simulink model "Multicopter_vPC"  (R2017b)
settings: Solver=ode4  StartTime=0.0  StopTime=inf  FixedStep=0.0002  RelTol=1e-3
values from neighbouring files (symbols this model uses):
  ModelFailBatt_CustomHovTime = 15    [Init.m]
  ModelFailBatt_isEnable = boolean(0)    [Init.m]
  ModelFailBatt_islowCapacity = boolean(0)    [Init.m]
  ModelFailBatt_isLowVoltage = boolean(0)    [Init.m]
  ModelFailBatt_isPowOff = boolean(0)    [Init.m]
  ModelFailBatt_isUseCustomHovTime = boolean(0)    [Init.m]
  ModelFailBatt_remainCapacityRatio = 0.2    [Init.m]
  ModelFailBatt_remainVoltageRatio = 0.5    [Init.m]
  ModelFailEnable = boolean(0)    [Init.m]
  ModelFailLoad_isEnable = boolean(0)    [Init.m]
  ModelFailLoad_isLoadFall = boolean(0)    [Init.m]
  ModelFailLoad_isLoadLeak = boolean(0)    [Init.m]
  ModelFailLoad_isLoadShift = boolean(0)    [Init.m]
  ModelFailLoad_LoadLeakRatioRate = 0    [Init.m]
  ModelFailLoad_loadMassRatio = 0    [Init.m]
  ModelFailLoad_LoadShiftXRatio = 0    [Init.m]
  ModelFailLoad_LoadShiftYRatio = 0    [Init.m]
  ModelFailLoad_LoadShiftZRatio = 0    [Init.m]
  ModelFailProp_isEnable = boolean(1)    [Init.m]
  ModelFailProp_PropEffRatioVec = ones(1,8)    [Init.m]
  ModelFailWind_ConstWindX = 0    [Init.m]
  ModelFailWind_ConstWindY = 0    [Init.m]
  ModelFailWind_ConstWindZ = 0    [Init.m]
  ModelFailWind_GustWindFreq = 0    [Init.m]
  ModelFailWind_GustWindStrength = 0    [Init.m]
  ModelFailWind_isConstWind = boolean(0)    [Init.m]
  ModelFailWind_isEnable = boolean(0)    [Init.m]
  ModelFailWind_isGustWind = boolean(0)    [Init.m]
  ModelFailWind_isSheerWind = boolean(0)    [Init.m]
  ModelFailWind_isTurbWind = boolean(0)    [Init.m]
  ModelFailWind_SheerWindDirec = 0    [Init.m]
  ModelFailWind_SheerWindStrength = 0    [Init.m]
  ModelFailWind_TurbWindDirec = 0    [Init.m]
  ModelFailWind_TurbWindStrength = 0    [Init.m]
  ModelInit_RPM = 0    [Init.m]
  ModelParam_BattHoverMinutes = 18    [Init.m]
  ModelParam_BattHoverThr = 0.609    [Init.m]
  ModelParam_envAltitude = -41.5260009765625    (= -41.5260009766)    [Init.m]
  ModelParam_GlobalNoiseGainSwitch = 0    [Init.m]
  ModelParam_GPSEphFinal = 0.3    [Init.m]
  ModelParam_GPSEpvFinal = 0.4    [Init.m]
  ModelParam_GPSFix3DFix = 3    [Init.m]
  ModelParam_GPSSatsVisible = 10    [Init.m]
  ModelParam_motorCr = 1148    [Init.m]
  ModelParam_motorJm = 0.0001287    [Init.m]
  ModelParam_motorMinThr = 0.05    [Init.m]
  ModelParam_motorT = 0.02    [Init.m]
  ModelParam_motorWb = -141.4    [Init.m]
  ModelParam_noiseBaroCoupleWithSpeed = 0    [Init.m]
  ModelParam_noiseGPSSampTime = 0.2    [Init.m]
  ModelParam_noisePowerIMU = 0    [Init.m]
  ModelParam_noisePowerOffGainAccel = 0.04    [Init.m]
  ModelParam_noisePowerOffGainAccelZ = 0.03    [Init.m]
  ModelParam_noisePowerOffGainGyro = 0.02    [Init.m]
  ModelParam_noisePowerOffGainGyroZ = 0.025    [Init.m]
  ModelParam_noisePowerOffGainMag = 0.02    [Init.m]
  ModelParam_noisePowerOffGainMagZ = 0.035    [Init.m]
  ModelParam_noisePowerOnGainAccel = 0.8    [Init.m]
  ModelParam_noisePowerOnGainAccelZ = 4.5    [Init.m]
  ModelParam_noisePowerOnGainGyro = 2    [Init.m]
  ModelParam_noisePowerOnGainGyroZ = 1    [Init.m]
  ModelParam_noisePowerOnGainMag = 0.025    [Init.m]
  ModelParam_noisePowerOnGainMagZ = 0.05    [Init.m]
  ModelParam_noiseSampleTimeAccel = 0.001    [Init.m]
  ModelParam_noiseSampleTimeGyro = 0.001    [Init.m]
  ModelParam_noiseSampleTimeMag = 0.01    [Init.m]
  ModelParam_noiseUpperBaro = 0    [Init.m]
  ModelParam_noiseUpperGPS = 0.5    [Init.m]
  ModelParam_noiseUpperWindBodyRatio = 0    [Init.m]
  ModelParam_noiseWindSampTime = 0.001    [Init.m]
  ModelParam_rotorCm = 1.779e-07    [Init.m]
  ModelParam_rotorCt = 1.105e-05    [Init.m]
  ModelParam_timeSampBaro = 0.01    [Init.m]
  ModelParam_uavCCm = [0.0035 0.0039 0.0034]    [Init.m]
  ModelParam_uavCd = 0.055    [Init.m]
  ModelParam_uavDearo = 0.12    [Init.m]
  ModelParam_uavJ = [ModelParam_uavJxx,0,0;     0,ModelParam_uavJyy,0;     0,0,ModelParam_uavJzz]    [Init.m]
  ModelParam_uavMass = 1.4    [Init.m]
  ModelParam_uavMotNumbs = int8(4)    [Init.m]
  ModelParam_uavR = 0.225    [Init.m]
  ModelParam_uavType = int8(3)    [Init.m]
undefined symbols (not defined in the file or in its folder): d_i, Earth, F, h_i, Light, MIL, ModelParam_GPSEphInitial, ModelParam_GPSEphTimeConstant, ModelParam_GPSEpvInitial, ModelParam_GPSEpvTimeConstant, ModelParam_noiseLowPassFilterCoeAccel, ModelParam_noiseLowPassFilterCoeGyro, ModelParam_timeSamp, Moderate, Newton, Raphson, WGS84
libraries: simulink x12, aerolibasang x4, aerolibwind2 x3, aerolibtransform2 x3, sharedtransform x3, aerolibutil x2, sharedutil x2, shared6dof x1, aerolibatmos2 x1, aerolibconvert2 x1, aerolibobsolete x1, aerolibnav x1
(part 2 of 3)

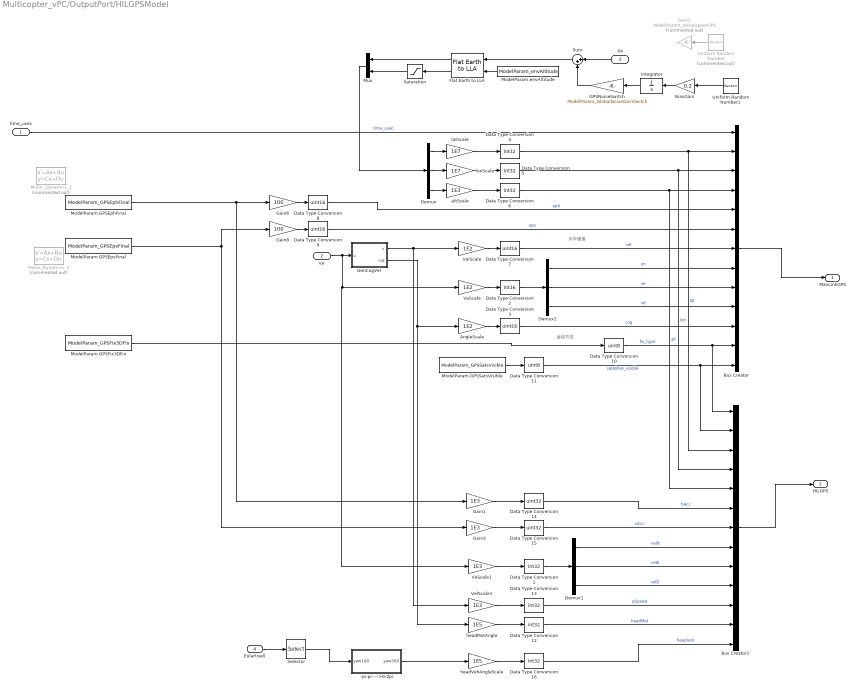
== system Multicopter_vPC/OutputPort/HILGPSModel ==
  note: 水平速度
  note: 运动方位
  time_usec : Inport
  Ve : Inport  Port=2
  Xe : Inport  Port=3
  Eular(rad) : Inport  Port=4
  -pi-pi---->0-2pi : MATLAB Function  TreatAsAtomicUnit=on
  AngleScale : Gain  Gain=1E2
  BiasGain : Gain  Gain=0.2
  Bus Creator : BusCreator  Inputs=13  OutDataTypeStr=Bus: MavLinkGPS  NonVirtualBus=on
  Bus Creator1 : BusCreator  Inputs=13  OutDataTypeStr=Bus: HILGPS  NonVirtualBus=on
  Data Type Conversion{1,4..6,12..13,16} (7 alike) : DataTypeConversion  OutDataTypeStr=int32
  Data Type Conversion10 : DataTypeConversion  OutDataTypeStr=uint8
  Data Type Conversion11 : DataTypeConversion  OutDataTypeStr=uint8
  Data Type Conversion14 : DataTypeConversion  OutDataTypeStr=uint32
  Data Type Conversion15 : DataTypeConversion  OutDataTypeStr=uint32
  Data Type Conversion2 : DataTypeConversion  OutDataTypeStr=int16
  Data Type Conversion{3,7..9} (4 alike) : DataTypeConversion  OutDataTypeStr=uint16
  Demux : Demux  Outputs=3
  Demux1 : Demux  Outputs=3
  Demux2 : Demux  Outputs=3
  Flat Earth to LLA : aerolibtransform2/Flat Earth to LLA  units=Metric (MKS)  ptype=Earth (WGS84)  F=1/298.257223563  R=6378137  LL0=ModelParam_GPSLatLong  psi=0
  GPSNoiseSwitch : Gain  Gain=ModelParam_GlobalNoiseGainSwitch
  Gain1 : Gain  Gain=1E3
  Gain2 : Gain  Commented=on  Gain=ModelParam_noiseUpperGPS
  Gain3 : Gain  Gain=1E3
  Gain6 : Gain  Gain=100
  Gain8 : Gain  Gain=100
  GenCogVel : MATLAB Function  TreatAsAtomicUnit=on
  Integrator : Integrator
  ModelParam.GPSEphFinal : Constant  Value=ModelParam_GPSEphFinal
  ModelParam.GPSEpvFinal : Constant  Value=ModelParam_GPSEpvFinal
  ModelParam.GPSFix3DFix : Constant  Value=ModelParam_GPSFix3DFix
  ModelParam.GPSSatsVisible : Constant  Value=ModelParam_GPSSatsVisible
  ModelParam.envAltitude : Constant  Value=ModelParam_envAltitude
  Motor_Dynamics_1 : StateSpace  Commented=on  A=-1/ModelParam_GPSEphTimeConstant  C=1/ModelParam_GPSEphTimeConstant  D=0  InitialCondition=ModelParam_GPSEphInitial*ModelParam_GPSEphTimeConstant
  Motor_Dynamics_2 : StateSpace  Commented=on  A=-1/ModelParam_GPSEpvTimeConstant  C=1/ModelParam_GPSEpvTimeConstant  D=0  InitialCondition=ModelParam_GPSEpvInitial*ModelParam_GPSEpvTimeConstant
  Mux : Mux  Inputs=2
  Saturation : Saturate  UpperLimit=100000  LowerLimit=0
  Selector : Selector  InputPortWidth=3  IndexOptions=Index vector (dialog)  Indices=[3]  OutputSizes=1
  Sum : Sum  Inputs=|++
  Uniform Random Number : UniformRandomNumber  Commented=on  Minimum=[-1,-1,-3]  Maximum=[1,1,3]  Seed=[14524,7875,698]  SampleTime=ModelParam_timeSamp
  Uniform Random Number1 : UniformRandomNumber  Minimum=[-1,-1,-1]  Maximum=[1,1,1]  Seed=[1452,787,69]  SampleTime=ModelParam_noiseGPSSampTime
  VeScale : Gain  Gain=1E2
  VeScale1 : Gain  Gain=1E3
  VelScale : Gain  Gain=1E2
  VelScale1 : Gain  Gain=1E3
  altScale : Gain  Gain=1E3
  headMotAngle : Gain  Gain=1E5
  headVehAngleScale : Gain  Gain=1E5
  latScale : Gain  Gain=1E7
  lonScale : Gain  Gain=1E7
  MavLinkGPS : Outport
  HILGPS : Outport  Port=2
  wires:
  Data Type Conversion16/1 -> Bus Creator1/13  "headVeh"
  headVehAngleScale/1 -> Data Type Conversion16/1
  Data Type Conversion12/1 -> Bus Creator1/12  "headMot"
  Data Type Conversion13/1 -> Bus Creator1/11  "gSpeed"
  Demux1/3 -> Bus Creator1/10  "velD"
  Demux1/2 -> Bus Creator1/9  "velE"
  Demux1/1 -> Bus Creator1/8  "velN"
  Data Type Conversion1/1 -> Demux1/1
  headMotAngle/1 -> Data Type Conversion12/1
  Data Type Conversion15/1 -> Bus Creator1/7  "vAcc"
  Data Type Conversion14/1 -> Bus Creator1/6  "hAcc"
  Gain3/1 -> Data Type Conversion15/1
  Gain1/1 -> Data Type Conversion14/1
  VeScale1/1 -> Data Type Conversion1/1
  VelScale1/1 -> Data Type Conversion13/1
  Data Type Conversion8/1 -> Bus Creator/5  "eph"
  Gain8/1 -> Data Type Conversion9/1
  Gain6/1 -> Data Type Conversion8/1
  Data Type Conversion9/1 -> Bus Creator/6  "epv"
  time_usec/1 -> Bus Creator/1  "time_usec"
  latScale/1 -> Data Type Conversion4/1
  lonScale/1 -> Data Type Conversion5/1
  altScale/1 -> Data Type Conversion6/1
  Data Type Conversion4/1 -> Bus Creator/2, Bus Creator1/3  "lat"
  Data Type Conversion5/1 -> Bus Creator/3, Bus Creator1/4  "lon"
  Data Type Conversion6/1 -> Bus Creator/4, Bus Creator1/5  "alt"
  Demux2/1 -> Bus Creator/8  "vn"
  Demux2/2 -> Bus Creator/9  "ve"
  Demux2/3 -> Bus Creator/10  "vd"
  VeScale/1 -> Data Type Conversion2/1
  Data Type Conversion2/1 -> Demux2/1
  VelScale/1 -> Data Type Conversion7/1
  Data Type Conversion7/1 -> Bus Creator/7  "vel"
  AngleScale/1 -> Data Type Conversion3/1
  Data Type Conversion3/1 -> Bus Creator/11  "cog"
  Data Type Conversion11/1 -> Bus Creator/13, Bus Creator1/2  "satellites_visible"
  Data Type Conversion10/1 -> Bus Creator/12, Bus Creator1/1  "fix_type"
  ModelParam.GPSSatsVisible/1 -> Data Type Conversion11/1
  Flat Earth to LLA/2 -> Saturation/1
  Saturation/1 -> Mux/2
  ModelParam.envAltitude/1 -> Flat Earth to LLA/2
  Xe/1 -> Sum/1
  Flat Earth to LLA/1 -> Mux/1
  Demux/1 -> latScale/1
  Demux/2 -> lonScale/1
  Demux/3 -> altScale/1
  Uniform Random Number/1 -> Gain2/1
  Sum/1 -> Flat Earth to LLA/1
  Uniform Random Number1/1 -> BiasGain/1
  Integrator/1 -> GPSNoiseSwitch/1
  BiasGain/1 -> Integrator/1
  Mux/1 -> Demux/1
  ModelParam.GPSEphFinal/1 -> Gain1/1, Gain6/1
  ModelParam.GPSEpvFinal/1 -> Gain8/1, Gain3/1
  ModelParam.GPSFix3DFix/1 -> Data Type Conversion10/1
  Ve/1 -> VeScale1/1, VeScale/1, GenCogVel/1(u)
  GenCogVel/1(v) -> VelScale/1, VelScale1/1
  GenCogVel/2(cot) -> AngleScale/1, headMotAngle/1
  Eular(rad)/1 -> Selector/1
  GPSNoiseSwitch/1 -> Sum/2
  Bus Creator/1 -> MavLinkGPS/1
  Bus Creator1/1 -> HILGPS/1
  -pi-pi---->0-2pi/1(yaw360) -> headVehAngleScale/1
  Selector/1 -> -pi-pi---->0-2pi/1(yaw180)

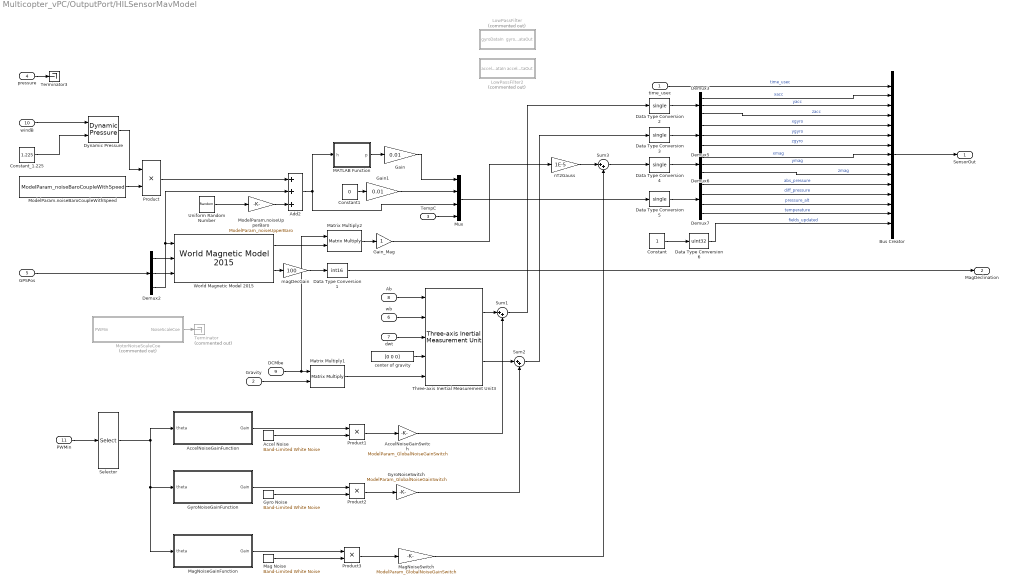
== system Multicopter_vPC/OutputPort/HILSensorMavModel ==
  time_usec : Inport
  Gravity : Inport  Port=2
  TempC : Inport  Port=3
  pressure : Inport  Port=4
  GPSPos : Inport  Port=5
  wb : Inport  Port=6
  dwt : Inport  Port=7
  Ab : Inport  Port=8
  DCMbe : Inport  Port=9
  windB : Inport  Port=10
  PWMin : Inport  Port=11
  Accel Noise : simulink/Sources/Band-Limited White Noise  Cov=ModelParam_noisePowerAccel  Ts=ModelParam_noiseSampleTimeAccel  seed=[411144,1416,71144]
  AccelNoiseGainFunction : MATLAB Function  TreatAsAtomicUnit=on
  AccelNoiseGainSwitch : Gain  Gain=ModelParam_GlobalNoiseGainSwitch
  Add2 : Sum  Inputs=+++
  Bus Creator : BusCreator  Inputs=15  OutDataTypeStr=Bus: MavLinkSensor  NonVirtualBus=on
  Constant : Constant
  Constant1 : Constant  Value=0
  Constant_1.225 : Constant  Value=1.225
  Data Type Conversion1 : DataTypeConversion  OutDataTypeStr=int16
  Data Type Conversion{2..5} (4 alike) : DataTypeConversion  OutDataTypeStr=single
  Data Type Conversion6 : DataTypeConversion  OutDataTypeStr=uint32
  Demux{2..3,5..6} (4 alike) : Demux  Outputs=3
  Demux7 : Demux
  Dynamic Pressure : aerolibasang/Dynamic Pressure
  Gain : Gain  Gain=0.01
  Gain1 : Gain  Gain=0.01
  Gain_Mag : Gain
  Gyro Noise : simulink/Sources/Band-Limited White Noise  Cov=ModelParam_noisePowerGyro  Ts=ModelParam_noiseSampleTimeGyro  seed=[111,116,144]
  GyroNoiseGainFunction : MATLAB Function  TreatAsAtomicUnit=on
  GyroNoiseSwitch : Gain  Gain=ModelParam_GlobalNoiseGainSwitch
  LowPassFilter : Subsystem  Commented=on
  LowPassFilter2 : Subsystem  Commented=on
  MATLAB Function : MATLAB Function  TreatAsAtomicUnit=on
  Mag Noise : simulink/Sources/Band-Limited White Noise  Cov=ModelParam_noisePowerMag  Ts=ModelParam_noiseSampleTimeMag  seed=[114,11699,999144]
  MagNoiseGainFunction : MATLAB Function  TreatAsAtomicUnit=on
  MagNoiseSwitch : Gain  Gain=ModelParam_GlobalNoiseGainSwitch
  Matrix Multiply1 : Product  Multiplication=Matrix(*)
  Matrix Multiply2 : Product  Multiplication=Matrix(*)
  ModelParam.noiseBaroCoupleWithSpeed : Constant  Value=ModelParam_noiseBaroCoupleWithSpeed
  ModelParam.noiseUpperBaro : Gain  Gain=ModelParam_noiseUpperBaro
  MotorNoiseScaleCoe : MATLAB Function  Commented=on  TreatAsAtomicUnit=on
  Mux : Mux
  Product{,1..3} (4 alike) : Product
  Selector : Selector  InputPortWidth=8  IndexOptions=Index vector (dialog)  Indices=[1]  OutputSizes=1
  Sum1 : Sum  Inputs=|++
  Sum2 : Sum  Inputs=|++
  Sum3 : Sum  Inputs=|++
  Terminator : Terminator  Commented=on
  Terminator3 : Terminator
  Three-axis Inertial Measurement Unit3 : aerolibnav/Three-axis Inertial Measurement Unit  units=Metric (MKS)  imu=[0 0 0]  i_Ts=0  dtype_a=on  w_a=190  z_a=0.707  a_sf_cc=[1 0 0; 0 1 0; 0 0 1]  a_bias=[0 0 0]  a_sat="[-160  -160  -160 160 160 160]"  dtype_g=on  w_g=190  z_g=0.707  g_sf_cc=[1 0 0; 0 1 0; 0 0 1]  g_bias=[0 0 0]  g_sens=[0 0 0]  g_sat="[-4.36  -4.36  -4.36 4.36 4.36 4.36]"  i_rand=off  i_seeds=[23093 23094 23095 23096 23097 23098]  i_pow=ModelParam_noisePowerIMU*[0.0000005 0.0000005 0.0000005 0.000000002 0.000000002 0.000000002]
  Uniform Random Number : UniformRandomNumber  Seed=15634  SampleTime=ModelParam_timeSampBaro
  World Magnetic Model 2015 : aerolibgravity2/World Magnetic Model 2015  units=Metric (MKS)  time_in=off  month=November  day=3  year=2017  action=Error  h_out=off  dec_out=on  inc_out=off  ti_out=off
      settings: SourceProductName=Aerospace Blockset  SourceProductBaseCode=AE
  center of gravity : Constant  Value=[0 0 0]
  magDecGain : Gain  Gain=100
  nT2Gauss : Gain  Gain=1E-5
  SensorOut : Outport
  MagDeclination : Outport  Port=2
  wires:
  center of gravity/1 -> Three-axis Inertial Measurement Unit3/4
  Sum1/1 -> Data Type Conversion2/1
  Sum2/1 -> Data Type Conversion3/1
  Sum3/1 -> Data Type Conversion4/1
  Matrix Multiply2/1 -> Gain_Mag/1
  magDecGain/1 -> Data Type Conversion1/1
  World Magnetic Model 2015/2 -> magDecGain/1
  ModelParam.noiseUpperBaro/1 -> Add2/3
  Product/1 -> Add2/1
  Dynamic Pressure/1 -> Product/1
  ModelParam.noiseBaroCoupleWithSpeed/1 -> Product/2
  Constant_1.225/1 -> Dynamic Pressure/2
  windB/1 -> Dynamic Pressure/1
  Uniform Random Number/1 -> ModelParam.noiseUpperBaro/1
  dwt/1 -> Three-axis Inertial Measurement Unit3/3
  Gain_Mag/1 -> nT2Gauss/1
  Constant1/1 -> Gain1/1
  pressure/1 -> Terminator3/1
  MATLAB Function/1(p) -> Gain/1
  Add2/1 -> MATLAB Function/1(h), Mux/3
  Demux2/3 -> World Magnetic Model 2015/1, Add2/2
  Demux2/2 -> World Magnetic Model 2015/3
  Demux2/1 -> World Magnetic Model 2015/2
  Matrix Multiply1/1 -> Three-axis Inertial Measurement Unit3/5
  DCMbe/1 -> Matrix Multiply2/1, Matrix Multiply1/1
  Gravity/1 -> Matrix Multiply1/2
  Gain1/1 -> Mux/2
  Gain/1 -> Mux/1
  Data Type Conversion6/1 -> Bus Creator/15  "fields_updated"
  Constant/1 -> Data Type Conversion6/1
  time_usec/1 -> Bus Creator/1  "time_usec"
  GPSPos/1 -> Demux2/1
  Demux7/2 -> Bus Creator/12  "diff_pressure"
  Demux7/3 -> Bus Creator/13  "pressure_alt"
  Demux6/2 -> Bus Creator/9  "ymag"
  Demux6/3 -> Bus Creator/10  "zmag"
  TempC/1 -> Mux/4
  Mux/1 -> Data Type Conversion5/1
  Demux7/1 -> Bus Creator/11  "abs_pressure"
  Demux5/2 -> Bus Creator/6  "ygyro"
  Demux6/1 -> Bus Creator/8  "xmag"
  Demux5/3 -> Bus Creator/7  "zgyro"
  Demux7/4 -> Bus Creator/14  "temperature"
  World Magnetic Model 2015/1 -> Matrix Multiply2/2
  Demux3/1 -> Bus Creator/2  "xacc"
  Demux3/2 -> Bus Creator/3  "yacc"
  Demux5/1 -> Bus Creator/5  "xgyro"
  Demux3/3 -> Bus Creator/4  "zacc"
  PWMin/1 -> Selector/1
  Ab/1 -> Three-axis Inertial Measurement Unit3/1
  wb/1 -> Three-axis Inertial Measurement Unit3/2
  MotorNoiseScaleCoe/1(NoiseScaleCoe) -> Terminator/1
  Selector/1 -> MagNoiseGainFunction/1(theta), GyroNoiseGainFunction/1(theta), AccelNoiseGainFunction/1(theta)
  AccelNoiseGainFunction/1(Gain) -> Product1/1
  GyroNoiseGainFunction/1(Gain) -> Product2/1
  Product1/1 -> AccelNoiseGainSwitch/1
  Product2/1 -> GyroNoiseSwitch/1
  Mag Noise/1 -> Product3/2
  nT2Gauss/1 -> Sum3/1
  Product3/1 -> MagNoiseSwitch/1
  MagNoiseGainFunction/1(Gain) -> Product3/1
  GyroNoiseSwitch/1 -> Sum2/2
  AccelNoiseGainSwitch/1 -> Sum1/2
  MagNoiseSwitch/1 -> Sum3/2
  Data Type Conversion2/1 -> Demux3/1
  Data Type Conversion3/1 -> Demux5/1
  Data Type Conversion4/1 -> Demux6/1
  Data Type Conversion5/1 -> Demux7/1
  Bus Creator/1 -> SensorOut/1
  Data Type Conversion1/1 -> MagDeclination/1
  Three-axis Inertial Measurement Unit3/1 -> Sum1/1
  Three-axis Inertial Measurement Unit3/2 -> Sum2/1
  Accel Noise/1 -> Product1/2
  Gyro Noise/1 -> Product2/2

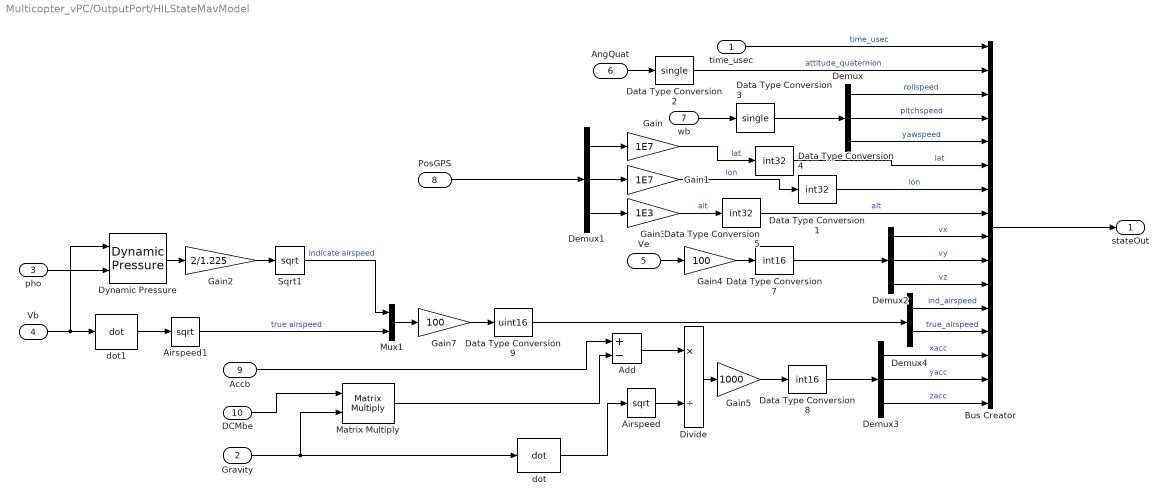
== system Multicopter_vPC/OutputPort/HILStateMavModel ==
  time_usec : Inport
  Gravity : Inport  Port=2
  pho : Inport  Port=3
  Vb : Inport  Port=4
  Ve : Inport  Port=5
  AngQuat : Inport  Port=6
  wb : Inport  Port=7
  PosGPS : Inport  Port=8
  Accb : Inport  Port=9
  DCMbe : Inport  Port=10
  Add : Sum  Inputs=+-
  Airspeed : Sqrt  AlgorithmType=Newton-Raphson  SaturateOnIntegerOverflow=on
  Airspeed1 : Sqrt  AlgorithmType=Newton-Raphson  SaturateOnIntegerOverflow=on
  Bus Creator : BusCreator  Inputs=16  OutDataTypeStr=Bus: MavLinkStateQuat  NonVirtualBus=on
  Data Type Conversion1 : DataTypeConversion  OutDataTypeStr=int32
  Data Type Conversion2 : DataTypeConversion  OutDataTypeStr=single
  Data Type Conversion3 : DataTypeConversion  OutDataTypeStr=single
  Data Type Conversion4 : DataTypeConversion  OutDataTypeStr=int32
  Data Type Conversion5 : DataTypeConversion  OutDataTypeStr=int32
  Data Type Conversion7 : DataTypeConversion  OutDataTypeStr=int16
  Data Type Conversion8 : DataTypeConversion  OutDataTypeStr=int16
  Data Type Conversion9 : DataTypeConversion  OutDataTypeStr=uint16
  Demux{,1..3} (4 alike) : Demux  Outputs=3
  Demux4 : Demux  Outputs=2
  Divide : Product  Inputs=*/
  Dynamic Pressure : aerolibasang/Dynamic Pressure
  Gain : Gain  Gain=1E7
  Gain1 : Gain  Gain=1E7
  Gain2 : Gain  Gain=2/1.225
  Gain3 : Gain  Gain=1E3
  Gain4 : Gain  Gain=100
  Gain5 : Gain  Gain=1000
  Gain7 : Gain  Gain=100
  Matrix Multiply : Product  Multiplication=Matrix(*)
  Mux1 : Mux  Inputs=2
  Sqrt1 : Sqrt  SaturateOnIntegerOverflow=on
  dot : aerolibasang/Incidence, Sideslip, & Airspeed/dot
      settings: SourceProductName=Aerospace Blockset  SourceProductBaseCode=AE
  dot1 : aerolibasang/Incidence, Sideslip, & Airspeed/dot
      settings: SourceProductName=Aerospace Blockset  SourceProductBaseCode=AE
  stateOut : Outport
  wires:
  Sqrt1/1 -> Mux1/1  "indicate airspeed"
  Gain2/1 -> Sqrt1/1
  Dynamic Pressure/1 -> Gain2/1
  time_usec/1 -> Bus Creator/1  "time_usec"
  Vb/1 -> dot1/1, Dynamic Pressure/1
  AngQuat/1 -> Data Type Conversion2/1
  Ve/1 -> Gain4/1
  Accb/1 -> Add/1
  wb/1 -> Data Type Conversion3/1
  Gravity/1 -> dot/1, Matrix Multiply/2
  Airspeed1/1 -> Mux1/2  "true airspeed"
  Mux1/1 -> Gain7/1
  Demux4/1 -> Bus Creator/12  "ind_airspeed"
  Demux4/2 -> Bus Creator/13  "true_airspeed"
  Demux3/3 -> Bus Creator/16  "zacc"
  Demux3/2 -> Bus Creator/15  "yacc"
  Demux3/1 -> Bus Creator/14  "xacc"
  Airspeed/1 -> Divide/2
  Gain5/1 -> Data Type Conversion8/1
  Divide/1 -> Gain5/1
  Demux2/3 -> Bus Creator/11  "vz"
  Demux2/2 -> Bus Creator/10  "vy"
  Demux2/1 -> Bus Creator/9  "vx"
  Gain4/1 -> Data Type Conversion7/1
  Gain3/1 -> Data Type Conversion5/1  "alt"
  Gain1/1 -> Data Type Conversion1/1  "lon"
  Gain/1 -> Data Type Conversion4/1  "lat"
  Demux1/3 -> Gain3/1
  Demux1/2 -> Gain1/1
  Demux1/1 -> Gain/1
  Demux/3 -> Bus Creator/5  "yawspeed"
  Demux/2 -> Bus Creator/4  "pitchspeed"
  Demux/1 -> Bus Creator/3  "rollspeed"
  Data Type Conversion2/1 -> Bus Creator/2  "attitude_quaternion"
  pho/1 -> Dynamic Pressure/2
  Gain7/1 -> Data Type Conversion9/1
  dot1/1 -> Airspeed1/1
  dot/1 -> Airspeed/1
  Data Type Conversion3/1 -> Demux/1
  PosGPS/1 -> Demux1/1
  Data Type Conversion7/1 -> Demux2/1
  Data Type Conversion9/1 -> Demux4/1
  Data Type Conversion8/1 -> Demux3/1
  Data Type Conversion4/1 -> Bus Creator/6  "lat"
  Data Type Conversion1/1 -> Bus Creator/7  "lon"
  Data Type Conversion5/1 -> Bus Creator/8  "alt"
  Bus Creator/1 -> stateOut/1
  DCMbe/1 -> Matrix Multiply/1
  Matrix Multiply/1 -> Add/2
  Add/1 -> Divide/1

== system Multicopter_vPC/Actuator Model: Motor_ESC/MotorNonlinearDynamic1/Motor_Dynamics ==
  motor_rate_d : Inport
  ModelInit_RPM : Inport  Port=2
  motorT : Inport  Port=3
  Add : Sum  Inputs=+-
  Divide : Product  Inputs=*/
  Integrator : Integrator  InitialConditionSource=external
  motor_rate_act : Outport
  wires:
  motorT/1 -> Divide/2
  Integrator/1 -> Add/2, motor_rate_act/1  "x"
  Divide/1 -> Integrator/1  "drate/dt"
  motor_rate_d/1 -> Add/1
  ModelInit_RPM/1 -> Integrator/2
  Add/1 -> Divide/1

== system Multicopter_vPC/Actuator Model: Motor_ESC/MotorNonlinearDynamic2/Motor_Dynamics ==
  motor_rate_d : Inport
  ModelInit_RPM : Inport  Port=2
  motorT : Inport  Port=3
  Add : Sum  Inputs=+-
  Divide : Product  Inputs=*/
  Integrator : Integrator  InitialConditionSource=external
  motor_rate_act : Outport
  wires:
  Add/1 -> Divide/1
  ModelInit_RPM/1 -> Integrator/2
  motor_rate_d/1 -> Add/1
  Divide/1 -> Integrator/1  "drate/dt"
  Integrator/1 -> motor_rate_act/1, Add/2  "x"
  motorT/1 -> Divide/2

== system Multicopter_vPC/Actuator Model: Motor_ESC/MotorNonlinearDynamic3/Motor_Dynamics ==
  motor_rate_d : Inport
  ModelInit_RPM : Inport  Port=2
  motorT : Inport  Port=3
  Add : Sum  Inputs=+-
  Divide : Product  Inputs=*/
  Integrator : Integrator  InitialConditionSource=external
  motor_rate_act : Outport
  wires:
  motorT/1 -> Divide/2
  Integrator/1 -> Add/2, motor_rate_act/1  "x"
  Divide/1 -> Integrator/1  "drate/dt"
  motor_rate_d/1 -> Add/1
  ModelInit_RPM/1 -> Integrator/2
  Add/1 -> Divide/1

== system Multicopter_vPC/Actuator Model: Motor_ESC/MotorNonlinearDynamic4/Motor_Dynamics ==
  motor_rate_d : Inport
  ModelInit_RPM : Inport  Port=2
  motorT : Inport  Port=3
  Add : Sum  Inputs=+-
  Divide : Product  Inputs=*/
  Integrator : Integrator  InitialConditionSource=external
  motor_rate_act : Outport
  wires:
  Add/1 -> Divide/1
  ModelInit_RPM/1 -> Integrator/2
  motor_rate_d/1 -> Add/1
  Divide/1 -> Integrator/1  "drate/dt"
  Integrator/1 -> motor_rate_act/1, Add/2  "x"
  motorT/1 -> Divide/2

== system Multicopter_vPC/Actuator Model: Motor_ESC/MotorNonlinearDynamic5/Motor_Dynamics ==
  motor_rate_d : Inport
  ModelInit_RPM : Inport  Port=2
  motorT : Inport  Port=3
  Add : Sum  Inputs=+-
  Divide : Product  Inputs=*/
  Integrator : Integrator  InitialConditionSource=external
  motor_rate_act : Outport
  wires:
  motorT/1 -> Divide/2
  Integrator/1 -> Add/2, motor_rate_act/1  "x"
  Divide/1 -> Integrator/1  "drate/dt"
  motor_rate_d/1 -> Add/1
  ModelInit_RPM/1 -> Integrator/2
  Add/1 -> Divide/1

== system Multicopter_vPC/Actuator Model: Motor_ESC/MotorNonlinearDynamic6/Motor_Dynamics ==
  motor_rate_d : Inport
  ModelInit_RPM : Inport  Port=2
  motorT : Inport  Port=3
  Add : Sum  Inputs=+-
  Divide : Product  Inputs=*/
  Integrator : Integrator  InitialConditionSource=external
  motor_rate_act : Outport
  wires:
  Add/1 -> Divide/1
  ModelInit_RPM/1 -> Integrator/2
  motor_rate_d/1 -> Add/1
  Divide/1 -> Integrator/1  "drate/dt"
  Integrator/1 -> motor_rate_act/1, Add/2  "x"
  motorT/1 -> Divide/2

== system Multicopter_vPC/Actuator Model: Motor_ESC/MotorNonlinearDynamic7/Motor_Dynamics ==
  motor_rate_d : Inport
  ModelInit_RPM : Inport  Port=2
  motorT : Inport  Port=3
  Add : Sum  Inputs=+-
  Divide : Product  Inputs=*/
  Integrator : Integrator  InitialConditionSource=external
  motor_rate_act : Outport
  wires:
  motorT/1 -> Divide/2
  Integrator/1 -> Add/2, motor_rate_act/1  "x"
  Divide/1 -> Integrator/1  "drate/dt"
  motor_rate_d/1 -> Add/1
  ModelInit_RPM/1 -> Integrator/2
  Add/1 -> Divide/1

== system Multicopter_vPC/Actuator Model: Motor_ESC/MotorNonlinearDynamic8/Motor_Dynamics ==
  motor_rate_d : Inport
  ModelInit_RPM : Inport  Port=2
  motorT : Inport  Port=3
  Add : Sum  Inputs=+-
  Divide : Product  Inputs=*/
  Integrator : Integrator  InitialConditionSource=external
  motor_rate_act : Outport
  wires:
  Add/1 -> Divide/1
  ModelInit_RPM/1 -> Integrator/2
  motor_rate_d/1 -> Add/1
  Divide/1 -> Integrator/1  "drate/dt"
  Integrator/1 -> motor_rate_act/1, Add/2  "x"
  motorT/1 -> Divide/2

== system Multicopter_vPC/Force and Moment Model/Propeller Model/Multicopter ==
  uavType : Inport
  MotorRads : Inport  Port=2
  uavR : Inport  Port=3
  uavDearo : Inport  Port=4
  Cm : Inport  Port=5
  Ct : Inport  Port=6
  Jm : Inport  Port=7
  wb : Inport  Port=8
  Action Port : ActionPort  InitializeStates=reset
  For Iterator Subsystem : Subsystem  TreatAsAtomicUnit=on
  Gain : Gain  Gain=-1
  Vector Concatenate : Concatenate
  Vector Concatenate1 : Concatenate  NumInputs=3  Mode=Multidimensional array
  uavTypeDefine : MATLAB Function  TreatAsAtomicUnit=on
  Fb : Outport
  Mb : Outport  Port=2
  wires:
  wb/1 -> For Iterator Subsystem/2(wb)
  uavR/1 -> Vector Concatenate/1
  uavDearo/1 -> Gain/1
  Gain/1 -> Vector Concatenate/2
  Vector Concatenate/1 -> For Iterator Subsystem/4(motorPositionVector)
  MotorRads/1 -> For Iterator Subsystem/5(motorOmegaVector)
  Cm/1 -> For Iterator Subsystem/9(rotorCm)
  Ct/1 -> For Iterator Subsystem/8(rotorCt)
  Jm/1 -> For Iterator Subsystem/6(motorJ_RP)
  For Iterator Subsystem/2(Mb) -> Mb/1
  For Iterator Subsystem/1(Fb) -> Fb/1
  uavType/1 -> uavTypeDefine/1(uavType)
  uavTypeDefine/1(n_p) -> For Iterator Subsystem/1(n_p)
  uavTypeDefine/5(motorRotateDirectionVector) -> For Iterator Subsystem/7(motorRotateDirectionVector)
  uavTypeDefine/4(motorPsiVector) -> Vector Concatenate1/3
  uavTypeDefine/3(motorThetaVector) -> Vector Concatenate1/2
  uavTypeDefine/2(motorPhiVector) -> Vector Concatenate1/1
  Vector Concatenate1/1 -> For Iterator Subsystem/3(motorEularMatrix)

== system Multicopter_vPC/Force and Moment Model/Propeller Model/Other Vehicle Types ==
  MotorRads : Inport
  Action Port : ActionPort  InitializeStates=reset
  Constant : Constant  Value=[0,0,0]
  Constant1 : Constant  Value=[0,0,0]
  Terminator : Terminator
  Fb : Outport
  Mb : Outport  Port=2
  wires:
  Constant/1 -> Fb/1
  Constant1/1 -> Mb/1
  MotorRads/1 -> Terminator/1

== system Multicopter_vPC/OutputPort/HILSensorMavModel/LowPassFilter ==
  gyroDataIn : Inport
  Demux1 : Demux  Outputs=3
  Mux1 : Mux  Inputs=3
  x : TransferFcn  Denominator=[ModelParam_noiseLowPassFilterCoeGyro 1]
  y : TransferFcn  Denominator=[ModelParam_noiseLowPassFilterCoeGyro 1]
  z : TransferFcn  Denominator=[ModelParam_noiseLowPassFilterCoeGyro 1]
  gyroDataOut : Outport
  wires:
  Mux1/1 -> gyroDataOut/1
  z/1 -> Mux1/3
  x/1 -> Mux1/1
  Demux1/1 -> x/1
  y/1 -> Mux1/2
  gyroDataIn/1 -> Demux1/1
  Demux1/2 -> y/1
  Demux1/3 -> z/1

== system Multicopter_vPC/OutputPort/HILSensorMavModel/LowPassFilter2 ==
  accelDataIn : Inport
  Demux1 : Demux  Outputs=3
  Mux1 : Mux  Inputs=3
  x : TransferFcn  Denominator=[ModelParam_noiseLowPassFilterCoeAccel 1]
  y : TransferFcn  Denominator=[ModelParam_noiseLowPassFilterCoeAccel 1]
  z : TransferFcn  Denominator=[ModelParam_noiseLowPassFilterCoeAccel 1]
  accelDataOut : Outport
  wires:
  Mux1/1 -> accelDataOut/1
  z/1 -> Mux1/3
  x/1 -> Mux1/1
  Demux1/1 -> x/1
  y/1 -> Mux1/2
  accelDataIn/1 -> Demux1/1
  Demux1/2 -> y/1
  Demux1/3 -> z/1

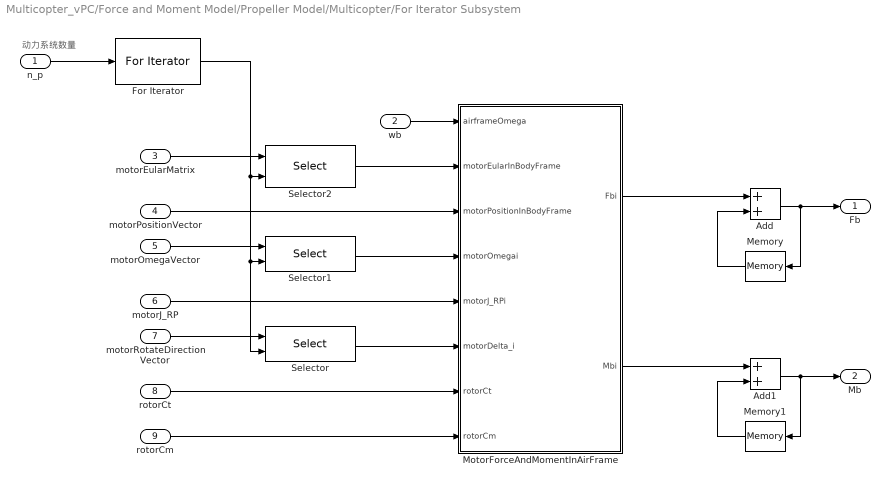
== system Multicopter_vPC/Force and Moment Model/Propeller Model/Multicopter/For Iterator Subsystem ==
  note: 动力系统数量
  n_p : Inport
  wb : Inport  Port=2
  motorEularMatrix : Inport  Port=3
  motorPositionVector : Inport  Port=4
  motorOmegaVector : Inport  Port=5
  motorJ_RP : Inport  Port=6
  motorRotateDirectionVector : Inport  Port=7
  rotorCt : Inport  Port=8
  rotorCm : Inport  Port=9
  Add : Sum
  Add1 : Sum
  For Iterator : ForIterator  ResetStates=reset  IterationSource=external
  Memory : Memory  InitialCondition=[0;0;0]  InheritSampleTime=on
  Memory1 : Memory  InitialCondition=[0;0;0]  InheritSampleTime=on
  MotorForceAndMomentInAirFrame : Subsystem  mask(Multicopter_Force_and_Moment_Model){}
      mask help: 在模块上右键帮助,查看帮助文档
      mask Help: web('doc/Multicopter_Force_and_Moment_Model.html')
  Selector : Selector  InputPortWidth=8  IndexOptions=Index vector (port)  Indices=[1 3]  OutputSizes=1
  Selector1 : Selector  InputPortWidth=8  IndexOptions=Index vector (port)  Indices=[1 3]  OutputSizes=1
  Selector2 : Selector  NumberOfDimensions=2  InputPortWidth=8  IndexOptions=Select all,Index vector (port)  Indices=[1 3],1  OutputSizes=1,1
  Fb : Outport
  Mb : Outport  Port=2
  wires:
  n_p/1 -> For Iterator/1
  wb/1 -> MotorForceAndMomentInAirFrame/1(airframeOmega)
  motorPositionVector/1 -> MotorForceAndMomentInAirFrame/3(motorPositionInBodyFrame)
  rotorCm/1 -> MotorForceAndMomentInAirFrame/8(rotorCm)
  rotorCt/1 -> MotorForceAndMomentInAirFrame/7(rotorCt)
  motorJ_RP/1 -> MotorForceAndMomentInAirFrame/5(motorJ_RPi)
  For Iterator/1 -> Selector2/2, Selector1/2, Selector/2
  motorRotateDirectionVector/1 -> Selector/1
  Selector/1 -> MotorForceAndMomentInAirFrame/6(motorDelta_i)
  Selector1/1 -> MotorForceAndMomentInAirFrame/4(motorOmegai)
  motorOmegaVector/1 -> Selector1/1
  Selector2/1 -> MotorForceAndMomentInAirFrame/2(motorEularInBodyFrame)
  motorEularMatrix/1 -> Selector2/1
  MotorForceAndMomentInAirFrame/1(Fbi) -> Add/1
  Memory/1 -> Add/2
  Add/1 -> Fb/1, Memory/1
  MotorForceAndMomentInAirFrame/2(Mbi) -> Add1/1
  Memory1/1 -> Add1/2
  Add1/1 -> Mb/1, Memory1/1

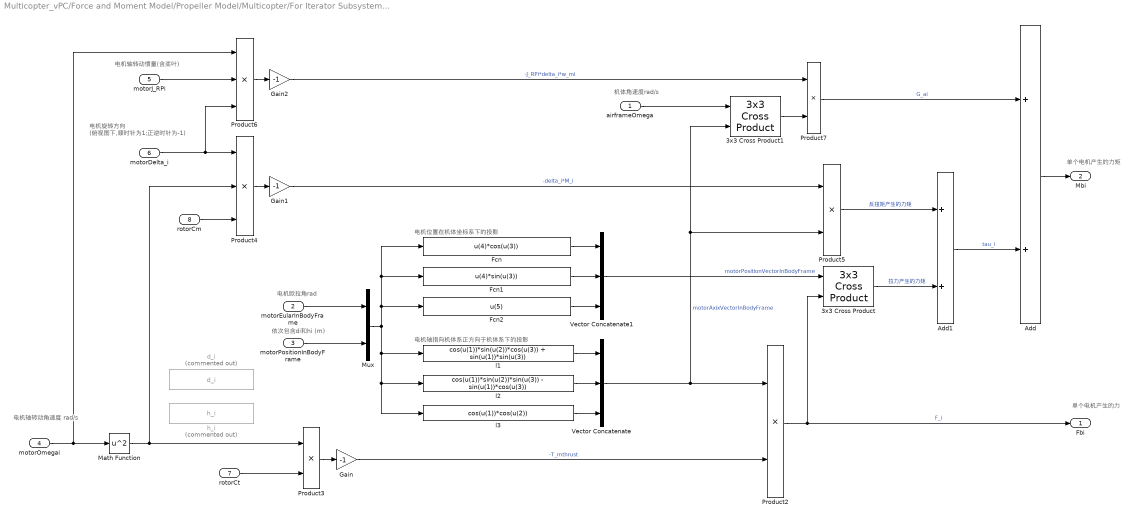
== system Multicopter_vPC/Force and Moment Model/Propeller Model/Multicopter/For Iterator Subsystem/MotorForceAndMomentInAirFrame ==
  note: 单个电机产生的力
  note: 单个电机产生的力矩
  note: 电机旋转方向
      | (俯视图下,顺时针为1;正逆时针为-1)
  note: 电机轴转动惯量(含桨叶)
  note: 机体角速度rad/s
  note: 电机轴转动角速度
      | rad/s
  note: 电机欧拉角rad
  note: 依次包含di和hi (m)
  note: 电机轴指向机体系正方向于机体系下的投影
  note: 电机位置在机体坐标系下的投影
  airframeOmega : Inport
  motorEularInBodyFrame : Inport  Port=2  PortDimensions=3
  motorPositionInBodyFrame : Inport  Port=3  PortDimensions=2
  motorOmegai : Inport  Port=4
  motorJ_RPi : Inport  Port=5
  motorDelta_i : Inport  Port=6
  rotorCt : Inport  Port=7
  rotorCm : Inport  Port=8
  3x3 Cross Product : sharedutil/3x3 Cross Product
      settings: SourceProductBaseCode=AE
  3x3 Cross Product1 : sharedutil/3x3 Cross Product
      settings: SourceProductBaseCode=AE
  Add : Sum  Inputs=2
  Add1 : Sum  Inputs=2
  Fcn : Fcn  Expr=u(4)*cos(u(3))
  Fcn1 : Fcn  Expr=u(4)*sin(u(3))
  Fcn2 : Fcn  Expr=u(5)
  Gain : Gain  Gain=-1
  Gain1 : Gain  Gain=-1
  Gain2 : Gain  Gain=-1
  Math Function : Math  Operator=square  SaturateOnIntegerOverflow=on
  Mux : Mux  Inputs=2
  Product{2..3,5,7} (4 alike) : Product
  Product4 : Product  Inputs=3
  Product6 : Product  Inputs=3
  Vector Concatenate : Concatenate  NumInputs=3
  Vector Concatenate1 : Concatenate  NumInputs=3
  d_i : Constant  Commented=on  Value=d_i
  h_i : Constant  Commented=on  Value=h_i
  l1 : Fcn  Expr=cos(u(1))*sin(u(2))*cos(u(3)) + sin(u(1))*sin(u(3))
  l2 : Fcn  Expr=cos(u(1))*sin(u(2))*sin(u(3)) - sin(u(1))*cos(u(3))
  l3 : Fcn  Expr=cos(u(1))*cos(u(2))
  Fbi : Outport
  Mbi : Outport  Port=2
  wires:
  Mux/1 -> Fcn2/1, Fcn1/1, Fcn/1, l3/1, l2/1, l1/1
  motorEularInBodyFrame/1 -> Mux/1
  Product3/1 -> Gain/1
  Gain/1 -> Product2/2  "-T_mthrust"
  rotorCt/1 -> Product3/2
  Math Function/1 -> Product4/2, Product3/1
  Product2/1 -> Fbi/1, 3x3 Cross Product/2  "F_i"
  Vector Concatenate/1 -> Product2/1, 3x3 Cross Product1/2, Product5/2  "motorAxixVectorInBodyFrame"
  motorOmegai/1 -> Product6/1, Math Function/1
  rotorCm/1 -> Product4/3
  l1/1 -> Vector Concatenate/1
  Gain1/1 -> Product5/1  "-delta_i*M_i"
  Gain2/1 -> Product7/1  "-J_RPi*delta_i*w_mi"
  Add1/1 -> Add/2  "tau_i"
  3x3 Cross Product/1 -> Add1/2  "拉力产生的力矩"
  l2/1 -> Vector Concatenate/2
  Fcn2/1 -> Vector Concatenate1/3
  Add/1 -> Mbi/1
  l3/1 -> Vector Concatenate/3
  Fcn1/1 -> Vector Concatenate1/2
  Vector Concatenate1/1 -> 3x3 Cross Product/1  "motorPositionVectorInBodyFrame"
  Fcn/1 -> Vector Concatenate1/1
  motorDelta_i/1 -> Product6/3, Product4/1
  Product5/1 -> Add1/1  "反扭矩产生的力矩"
  3x3 Cross Product1/1 -> Product7/2
  Product6/1 -> Gain2/1
  airframeOmega/1 -> 3x3 Cross Product1/1
  Product4/1 -> Gain1/1
  motorJ_RPi/1 -> Product6/2
  Product7/1 -> Add/1  "G_ai"
  motorPositionInBodyFrame/1 -> Mux/2

== matlab function Multicopter_vPC/Battery Model/MATLAB Function ==
  data: load input; time input; EffRatio output; hover_time input; hover_thr input; motorNumbs input; cell_voltage output; isEnable input; isUseCustomHovTime input; CustomHovTime input; isPowOff input; isLowVoltage input; remainVoltageRatio input; islowCapacity input; remainCapacityRatio input; remCapacity output
function [EffRatio, cell_voltage,remCapacity]= LiPo(load,time,hover_time,hover_thr,motorNumbs,isEnable,isUseCustomHovTime,CustomHovTime,isPowOff,isLowVoltage,remainVoltageRatio,islowCapacity,remainCapacityRatio)
%% battery model
%================================Constants=================================

delta_t = 0.01;
%max_current = 5.500;                % maximum current per motor             (A)
%aux_current = 0.100;                % current of auxillary components       (A)        
%capacity = 1.000;                   % LiPo current capacity                 (Ah)                                 
%cells = 2;                          % LiPo cell count

%==========================================================================

persistent discharge;
if isempty(discharge)
    discharge = 0;
end

persistent startTime;
if isempty(startTime)
    startTime = 0;
end

persistent reset;
if isempty(reset)
    reset = 0;
end

discharge_capacity=0;

% 低电量故障
if isEnable&&islowCapacity
   hover_time = hover_time*remainCapacityRatio;
   isUseCustomHovTime=false;
end


if isEnable&&~isUseCustomHovTime 
    capacity=1;
    
    if hover_time<0.01
        hover_time=0.01;
    end
    
    hover_current=1/(hover_time*1.4/60);
    current=0;
    for i=1:motorNumbs
        current=current+hover_current*(load(i)/hover_thr)^2;
    end
    aux_current=0.5;
    %current = sum(hover_current .* (load/hover_thr).^2) + aux_current;
    current =(current+aux_current)/double(motorNumbs);
    discharge = current * (delta_t / 3600) + discharge;
    discharge_capacity = discharge / capacity;    
end




%如果启用电池模型且使用自定义续航时间
if isEnable&&isUseCustomHovTime
      hover_time=CustomHovTime*1.4*60;
      if reset<0.5
         startTime=time;
         reset=1;
      end
      if hover_time<0.01
          hover_time=0.01;
      end
     discharge_capacity=(time-startTime)/hover_time;
else
    %使用默认的续航算法
    reset=0;
end


if discharge_capacity<0
    discharge_capacity=0;
end
if discharge_capacity>1
    discharge_capacity=1;
end


%电量与电压的曲线
if (0 <= discharge_capacity) && (discharge_capacity <=0.20)
    cell_voltage = -14.029*discharge_capacity^3 + 16.975*discharge_capacity^2 - 5.3339*discharge_capacity + 4.2;
elseif (0.20 < discharge_capacity) && (discharge_capacity < 0.70)
    cell_voltage = -0.2*discharge_capacity + 3.74;
else
    cell_voltage = -48*discharge_capacity^3 + 89.6*discharge_capacity^2 - 55.08*discharge_capacity + 14.716;
end

if cell_voltage < 0.5
    cell_voltage = 0;
end

% 电池失效故障
if isEnable&&isPowOff
     cell_voltage = 0; 
end

% 低电压故障
if isEnable&&isLowVoltage
    if remainVoltageRatio>1
        remainVoltageRatio=1;
    elseif remainVoltageRatio<0
        remainVoltageRatio=0;
    end
     cell_voltage = remainVoltageRatio*4.2;
end


%如果电池模型未启用，续航为无穷久，同时各个全局变量归零
if ~isEnable
    cell_voltage=4.2;
    discharge = 0;
    startTime = 0;
    reset = 0;
end

%效率矩阵
EffRatio=cell_voltage/4.2;
remCapacity=1-discharge_capacity;
%==========================================================================

== matlab function Multicopter_vPC/Force and Moment Model/Ground Model/Ground Model ==
  settings: updateMethod=DISCRETE
  data: mg input; wb input; Xe input; F1 output; Ve input; M1 output; Quet input; terrainZ input; landed output; takeoff output
function [F1,M1,landed,takeoff] = fcn(mg,wb,Xe,Ve,Quet,terrainZ)
% This is a ground model that can provides reaction force and reaction torque

% persistent z0;
% if isempty(z0)
%      z0=0;
% end

persistent takeoffFlag;
if isempty(takeoffFlag)
     takeoffFlag=int8(0);
end

persistent landFlag;
if isempty(landFlag)
     landFlag=int8(1);
end


z=Xe(3)-terrainZ;

 if (z<-0.3)&&(Ve(3)<-0.1)&&(takeoffFlag<0.5)
    takeoffFlag=int8(1);
    landFlag=int8(0);
 end
 
 if (z>-0.05)&&(Ve(3)>0.1)&&(landFlag<0.5)
    landFlag=int8(1);
    takeoffFlag=int8(0);
    %z0=terrainZ;
 end

takeoff = takeoffFlag;
landed = landFlag;


F1=[0;0;0];
M1=[0;0;0];

if z>=0
%     if z>=0.3
%         if Ve(3)>=5
%             F1(3)=-mg(3)-1000*Ve(3);
%         else
%             F1(3)=-mg(3)-500*z-100*Ve(3);  
%         end
%     elseif z>=0.1
%         if Ve(3)>=2
%             F1(3)=-mg(3)-100*Ve(3);
%         else
%             F1(3)=-mg(3)-50*z-100*Ve(3);  
%         end
%     else
%          if Ve(3)>=1
%             F1(3)=-mg(3)-50*Ve(3);
%         else
%             F1(3)=-mg(3)-5*z-50*Ve(3);  
%         end       
%     end
    if z<0.05
         F1(3)=-mg(3)-10*Ve(3); 
    elseif z<0.1
        F1(3)=-mg(3)-0.5*z-20*Ve(3); 
    else
         F1(3)=-mg(3)-1*z-50*Ve(3); 
    end

    
    F1(1)=-50*Ve(1);
    F1(2)=-50*Ve(2);
    M1=-200*[Quet(2);Quet(3);Quet(4)]-10*wb;
end

== matlab function Multicopter_vPC/Actuator Model: Motor_ESC/Propeller Fail model ==
  data: u input; y output; isEnable input; PropEffRatioVec input
function y = fcn(u, isEnable, PropEffRatioVec)
% This is a propeller failure model. PropEffRatioVec is a 1*8 vector 
% about propeller efficiency with the value range [0 1]. 

if isEnable
    y=PropEffRatioVec.*u;
else
    y = u;    
end

== matlab function Multicopter_vPC/OutputPort/HILGPSModel/-pi-pi---->0-2pi ==
  data: yaw180 input; yaw360 output
function yaw360 = fcn(yaw180)
%//rad
if yaw180>0
    yaw360 = yaw180;
else
    yaw360 = yaw180 +2*pi;
end

== matlab function Multicopter_vPC/OutputPort/HILSensorMavModel/MATLAB Function ==
  data: h input; p output
function p = fcn(h)
p=((1-h/0.3048/145366.45))^(1/0.190284)*101325;

== matlab function Multicopter_vPC/OutputPort/HILGPSModel/GenCogVel ==
  data: v output; u input; cot output
function [v,cot] = Ang360(u)
 cot=atan2d(u(2),u(1));
if cot<0
    cot=cot+360;
end

v=norm(u(1:2));

== matlab function Multicopter_vPC/Environment Model/MATLAB Function ==
  settings: updateMethod=DISCRETE
  data: t input; isGustWind input; gWind output; GustWindStrength input; GustWindFreq input; turb input
function gWind = GustWindModel(t,isGustWind,GustWindStrength,GustWindFreq,turb)

if(GustWindFreq<1)
    GustWindFreq=1;
end
timeVel=60/GustWindFreq;

vmax=GustWindStrength;

persistent t0;
if isempty(t0)
    t0=0;
end

persistent isInGust;
if isempty(isInGust)
    isInGust=0;
end

persistent t1;
if isempty(t1)
    t1=2;
end

persistent a;
if isempty(a)
    a=0.5;
end

persistent ang;
if isempty(ang)
    ang=pi/2;
end

persistent wlast;
if isempty(wlast)
    wlast=vmax*0.5;
end

persistent wNow;
if isempty(wNow)
    wNow=1.4*0.8*vmax;
end


if isGustWind&&isInGust<0.5
    t0=t;
    t1=timeVel*(3/4+1/2*rand(1));
    a=1/4+1/2*rand(1);
    ang=pi*2*rand(1);
    wlast=wNow;
    wNow=1.2*(rand(1)*0.5+0.5)*vmax;
    
    isInGust=1;
end

if ~isGustWind
    isInGust=0;
end

gWind=[0;0;0];

if(t<t0+t1*a)
    gWindMag=(wNow-wlast)/2*(1-cos((t-t0)/(t1*a)*pi))+wlast;
else
    gWindMag=wNow;
end

if abs(t-(t0+t1))<0.05
    rng(t*1000);
    t0=t;
    t1=timeVel*(3/4+1/2*rand(1));
    a=1/4+1/2*rand(1);
    ang=ang+0.1*pi*rand(1);
    wlast=wNow;
    wNow=1.2*(rand(1)*0.5+0.5)*vmax;
end

gWind(1)=gWindMag*cos(ang)*0.8+turb(1)*0.4;
gWind(2)=gWindMag*sin(ang)*0.8+turb(2)*0.4;
gWind(3)=turb(3)*0.4;

== matlab function Multicopter_vPC/Force and Moment Model/Ground Model/OnGroundFaceup ==
  data: EulerAng input; y output
function y = fcn(EulerAng)

targetRoll = 0;
% if cos(EulerAng(1))<0
%     targetRoll=pi;  
% end

targetPitch = 0;
% if cos(EulerAng(2))<0
%         targetPitch=pi;
% end
    
y = [targetRoll;targetPitch;EulerAng(3)];

== matlab function Multicopter_vPC/OutputPort/ZLimit ==
  data: zt input; xe input; Xee output
function Xee = fcn(zt,xe)
Xee=xe;
if Xee(3)>zt
    Xee(3)=zt;
end

== matlab function Multicopter_vPC/Environment Model/MATLAB Function1 ==
  data: isEnable input; wind output size=3; isConstWind input; isGustWind input; isTurbWind input; isSheerWind input; ConstWind input; GustWind input; TurbWind input; SheerWind input
function wind = WindFun(isEnable,isConstWind,isGustWind,isTurbWind,isSheerWind,ConstWind,GustWind,TurbWind,SheerWind)
wind=[0;0;0];
if isEnable
    if isConstWind
        wind=ConstWind;
    elseif isGustWind
        wind=GustWind;
    elseif isTurbWind
        wind=TurbWind;
    elseif isSheerWind
        wind=SheerWind;
    end
end

== matlab function Multicopter_vPC/OutputPort/Model Fail Assessment ==
  settings: updateMethod=DISCRETE
  data: ModelFailEnable input; landed input; FailInfo output; ve input; xe input; wb input; ang input
function FailInfo  = fcn(ModelFailEnable,landed,ve,xe,wb,ang)

persistent xTemp;
if isempty(xTemp)
     xTemp=zeros(8,1);
end

persistent kk;
if isempty(kk)
     kk=0;
end

persistent ss;
if isempty(ss)
     ss=zeros(6,1);
end

if ~ModelFailEnable&&(kk<0.5)
    xTemp=zeros(8,1);
    kk=0;
    ss=[xe;ang];
end

if ModelFailEnable&&~landed
    xTemp(1:4,1)=[norm(xe-ss(1:3,1));norm(ve);norm(ang-ss(4:6,1));norm(wb)];
    xTemp(5:8,1)= (xTemp(5:8,1)*kk+xTemp(1:4,1))/(kk+1);
    
    kk=kk+1;
end
%landed = int8(0);
 
FailInfo=xTemp;

== matlab function Multicopter_vPC/Fail Model/Model Failure ==
  settings: updateMethod=DISCRETE
  data: T input; uavMass input; uavR input; uavlostMass output; uavlostJ output; isEnable input; loadMassRatio input; isLoadFall input; isLoadShift input; LoadShiftXRatio input; LoadShiftYRatio input; LoadShiftZRatio input; isLoadLeak input; LoadLeakRatioRate input; dcm input; deltaM output
function [uavlostMass,uavlostJ,deltaM] = fcn(T,uavMass,uavR,isEnable,loadMassRatio,isLoadFall,isLoadShift,LoadShiftXRatio,LoadShiftYRatio,LoadShiftZRatio,isLoadLeak,LoadLeakRatioRate,dcm)
% This function aims to calculate the variation of mass and moment of
% inertia caused by model failure including LoadFall, LoadShift, and
% LoadLeak.

persistent tOld;
if isempty(tOld)  
   tOld=0;
end    

deltaM=[0;0;0];

if isEnable

    if isLoadFall
         uavlostMass=loadMassRatio*uavMass;
         uavlostJ=zeros(3,3); 
    elseif isLoadShift

        uavlostMass= 0;
        loadMoveMass= loadMassRatio*uavMass;

        X=uavR*LoadShiftXRatio;
        Y=uavR*LoadShiftYRatio;
        Z=uavR*LoadShiftZRatio;

        uavlostJxx= loadMoveMass*(Y^2+Z^2);
        uavlostJyy= loadMoveMass*(X^2+Z^2);
        uavlostJzz= loadMoveMass*(X^2+Y^2);
        uavlostJyz= loadMoveMass*Y*Z;
        uavlostJzx= loadMoveMass*Z*X;
        uavlostJxy= loadMoveMass*X*Y;
        uavlostJ=-[uavlostJxx,-uavlostJxy,-uavlostJzx;-uavlostJxy,uavlostJyy,-uavlostJyz;-uavlostJzx,-uavlostJyz,uavlostJzz];
        
        deltaF = dcm*loadMoveMass*[0;0;9.8];
        
        deltaM = cross([X;Y;Z],deltaF);     % 变化的力矩 

    elseif isLoadLeak    
        uavlostJ=zeros(3,3);
        loadmass0=loadMassRatio*uavMass;

        if tOld<0.01
           tOld=T;
        end 

        dt=T-tOld;

        LoadLeakRatio = LoadLeakRatioRate*dt;
        if LoadLeakRatio > 1
          LoadLeakRatio = 1;  
        end    
        uavlostMass = LoadLeakRatio*loadmass0;  
        
    else
        uavlostMass=0;
        uavlostJ=zeros(3,3);
    end

    if ~isLoadLeak    %reset
        tOld=0;
    end

else
     uavlostMass=0;
     uavlostJ=zeros(3,3);
     tOld=0;
 end

== matlab function Multicopter_vPC/Force and Moment Model/Propeller Model/Multicopter/uavTypeDefine ==
  data: uavType input; n_p output; motorPhiVector output; motorThetaVector output; motorPsiVector output; motorRotateDirectionVector output
function [n_p,motorPhiVector,motorThetaVector,motorPsiVector,motorRotateDirectionVector]  = fcn(uavType)
% -1: anticlockwise, 1: clockwise 
TypeMotorDirMatrix=[...
    [-1 -1 -1 0 0 0 0 0];... % Tri 3*1 X           Type1
    [1 1 1 0 0 0 0 0];...    % Tri 3*1 +            Type2
    [-1 -1 1 1 0 0 0 0];... % Quad 4*1 X        Type3
    [-1 -1 1 1 0 0 0 0];... % Quad 4*1 +        Type4
    [1 -1 1 -1 -1 1 0 0];... % Hex 6*1 X         Type5
    [1 -1 1 -1 -1 1 0 0];... % Hex 6*1 +         Type6
    [1 -1 1 -1 1 -1 0 0];... % HexCoa 3*2      Type7
    [1 1 -1 -1 -1 -1 1 1];... % Oct 8*1 X        Type8
    [1 1 -1 -1 -1 -1 1 1];... % Oct 8*1 +        Type9
    [1 -1 1 -1 1 -1 1 -1];... % OctCoa 4*2 X  Type10
    [-1 -1 1 1 0 0 0 0];... % Intel Aero          Type11
    [-1 -1 1 1 0 0 0 0];... % custom              Type12
];

TypeMotorPsiAngMatrix=[...
    [pi/3 pi -pi/3 0 0 0 0 0];...%Type1
    [pi/3 pi -pi/3 0 0 0 0 0];...%Type2
    [pi/4   pi/4+pi     pi/4+3*pi/2     pi/4+pi/2   0 0 0 0];...%Type3
    [pi/2 3*pi/2 0 pi 0 0 0 0];...%Type4
    [pi/2 3/2*pi 3/2*pi+pi/3 pi/2+pi/3 pi/2-pi/3 3/2*pi-pi/3 0 0];...%Type5
    [0 pi pi+pi/3 pi/3 -pi/3 pi-pi/3 0 0];...%Type6
    [pi/3 pi/3 pi pi -pi/3 -pi/3 0 0];...%Type7
    [pi/8 pi+pi/8 pi/8+pi/4 pi-pi/8 -pi/8 3/2*pi-pi/8 3/2*pi+pi/8 pi/2+pi/8];...%Type8
    [0 pi pi/4 3/4*pi -pi/4 pi+pi/4 3/2*pi pi/2];...%Type9
    [pi/4 -pi/4 pi+pi/4 pi-pi/4 -pi/4 pi/4 pi-pi/4 pi+pi/4];...%Type10
    [43*pi/180     223*pi/180      317*pi/180      137*pi/180     0 0 0 0];...%Type11  Intel Aero
    [pi/4   pi/4+pi     pi/4+3*pi/2     pi/4+pi/2   0 0 0 0];...%Type12  custom
];

TypeMotorThetaAngMatrix=[...
    [0 0 0 0 0 0 0 0];...%Type1
    [0 0 0 0 0 0 0 0];...%Type2
    [0 0 0 0 0 0 0 0];...%Type3
    [0 0 0 0 0 0 0 0];...%Type4
    [0 0 0 0 0 0 0 0];...%Type5
    [0 0 0 0 0 0 0 0];...%Type6
    [0 0 0 0 0 0 0 0];...%Type7
    [0 0 0 0 0 0 0 0];...%Type8
    [0 0 0 0 0 0 0 0];...%Type9
    [0 0 0 0 0 0 0 0];...%Type10
    [0 0 0 0 0 0 0 0];...%Type11
    [pi/4   pi/4    pi/4    pi/4    0 0 0 0];...%Type12
    ];
TypeMotorPhiAngMatrix=[...
    [0 0 0 0 0 0 0 0];...%Type1
    [0 0 0 0 0 0 0 0];...%Type2
    [0 0 0 0 0 0 0 0];...%Type3
    [0 0 0 0 0 0 0 0];...%Type4
    [0 0 0 0 0 0 0 0];...%Type5
    [0 0 0 0 0 0 0 0];...%Type6
    [0 0 0 0 0 0 0 0];...%Type7
    [0 0 0 0 0 0 0 0];...%Type8
    [0 0 0 0 0 0 0 0];...%Type9
    [0 0 0 0 0 0 0 0];...%Type10
    [0 0 0 0 0 0 0 0];...%Type11
    [0 0 0 0 0 0 0 0];...%Type12
];

TypeMotorNonVector=int8([3;3;4;4;6;6;6;8;8;8;4;4]);

if uavType<0||uavType>length(TypeMotorNonVector)
    uavType=int8(1);
end

motorRotateDirectionVector=TypeMotorDirMatrix(uavType,:);
motorPsiVector=TypeMotorPsiAngMatrix(uavType,:);
motorThetaVector=TypeMotorThetaAngMatrix(uavType,:);
motorPhiVector=TypeMotorPhiAngMatrix(uavType,:);
n_p = TypeMotorNonVector(uavType);

== matlab function Multicopter_vPC/OutputPort/HILSensorMavModel/AccelNoiseGainFunction ==
  data: theta input; Gain output; ModelParam_noisePowerOnGainAccel parameter; ModelParam_noisePowerOffGainAccel parameter; ModelParam_noisePowerOnGainAccelZ parameter; ModelParam_noisePowerOffGainAccelZ parameter
function Gain = fcn(theta, ModelParam_noisePowerOnGainAccel, ModelParam_noisePowerOffGainAccel,ModelParam_noisePowerOnGainAccelZ, ModelParam_noisePowerOffGainAccelZ)
%#codegen
if theta>0.1
Gain = [ModelParam_noisePowerOnGainAccel;ModelParam_noisePowerOnGainAccel;ModelParam_noisePowerOnGainAccelZ];
else
    Gain = [ModelParam_noisePowerOffGainAccel;ModelParam_noisePowerOffGainAccel;ModelParam_noisePowerOffGainAccelZ];
end

== matlab function Multicopter_vPC/OutputPort/HILSensorMavModel/GyroNoiseGainFunction ==
  data: theta input; Gain output; ModelParam_noisePowerOnGainGyro parameter; ModelParam_noisePowerOffGainGyro parameter; ModelParam_noisePowerOnGainGyroZ parameter; ModelParam_noisePowerOffGainGyroZ parameter
function Gain = fcn(theta, ModelParam_noisePowerOnGainGyro, ModelParam_noisePowerOffGainGyro, ModelParam_noisePowerOnGainGyroZ, ModelParam_noisePowerOffGainGyroZ)
%#codegen
if theta>0.1
    Gain = [ModelParam_noisePowerOnGainGyro;ModelParam_noisePowerOnGainGyro;ModelParam_noisePowerOnGainGyroZ];
else
    Gain = [ModelParam_noisePowerOffGainGyro;ModelParam_noisePowerOffGainGyro;ModelParam_noisePowerOffGainGyroZ];
end

== matlab function Multicopter_vPC/OutputPort/HILSensorMavModel/MagNoiseGainFunction ==
  data: theta input; Gain output; ModelParam_noisePowerOnGainMag parameter; ModelParam_noisePowerOffGainMag parameter; ModelParam_noisePowerOnGainMagZ parameter; ModelParam_noisePowerOffGainMagZ parameter
function Gain = fcn(theta, ModelParam_noisePowerOnGainMag, ModelParam_noisePowerOffGainMag, ModelParam_noisePowerOnGainMagZ, ModelParam_noisePowerOffGainMagZ)
%#codegen
if theta>0.1
    Gain = [ModelParam_noisePowerOnGainMag;ModelParam_noisePowerOnGainMag;ModelParam_noisePowerOnGainMagZ];
else
    Gain = [ModelParam_noisePowerOffGainMag;ModelParam_noisePowerOffGainMag;ModelParam_noisePowerOffGainMagZ];
end
